simulink model "test"  (R2022a)
settings: Solver=VariableStepAuto  StartTime=0.0  StopTime=30  RelTol=1e-3
values from neighbouring files (symbols this model uses):
  n = length(stations)    [ethernetHubMask.m]
undefined symbols (not defined in the file or in its folder): gateControl, m, networkselector
settings Model: Creator=lch  LastModifiedBy=lch

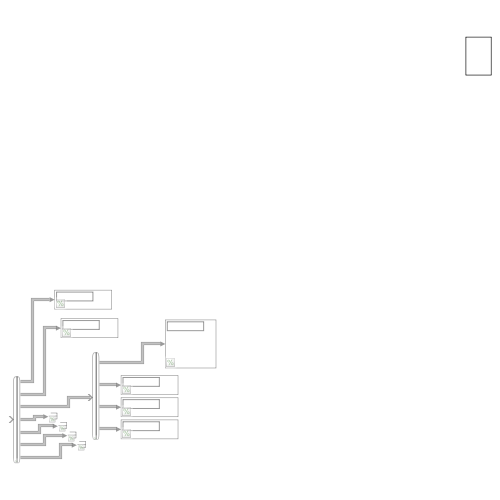
[thumbnail: Simulink's stored preview of the top-level diagram]
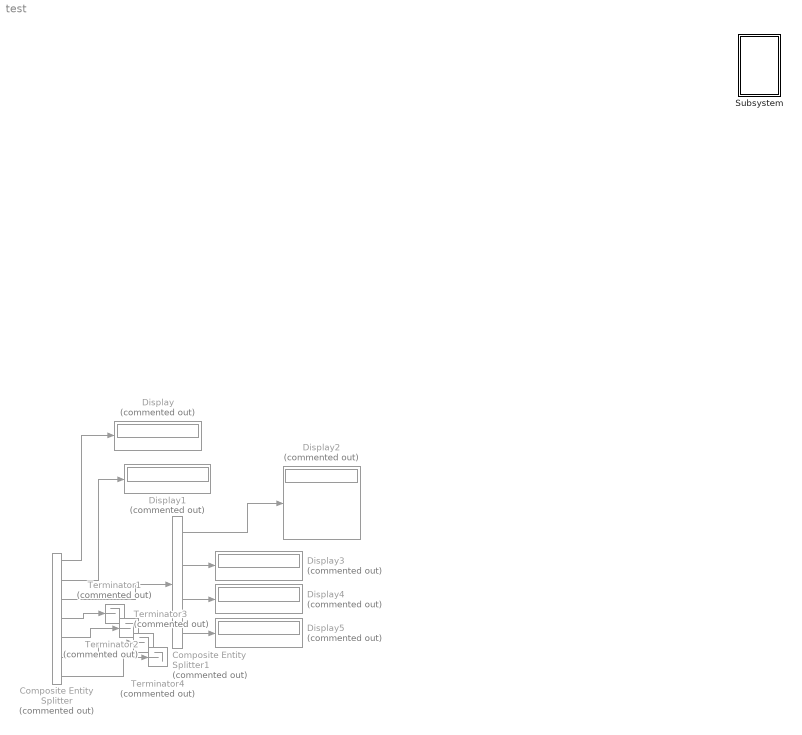
== system test ==
  Composite Entity Splitter : CompositeEntitySplitter  Commented=on  InputPortMessageModes=m  OutputPortMessageModes=m,m,m,m,m,m,m  NumberOutputPorts=7
      settings: OutputPortMap=o0,o1,o2,o3,o4,o5,o6
  Composite Entity Splitter1 : CompositeEntitySplitter  Commented=on  InputPortMessageModes=m  OutputPortMessageModes=m,m,m,m  NumberOutputPorts=4
      settings: OutputPortMap=o0,o1,o2,o3
  Display{,1..5} (6 alike) : Display  Commented=on
  Subsystem : Subsystem
  Terminator{1..4} (4 alike) : Terminator  Commented=on
  wires:
  Composite Entity Splitter/1 -> Display/1
  Composite Entity Splitter/2 -> Display1/1
  Composite Entity Splitter/3 -> Composite Entity Splitter1/1
  Composite Entity Splitter/4 -> Terminator1/1
  Composite Entity Splitter/5 -> Terminator2/1
  Composite Entity Splitter/6 -> Terminator3/1
  Composite Entity Splitter/7 -> Terminator4/1
  Composite Entity Splitter1/1 -> Display2/1
  Composite Entity Splitter1/2 -> Display3/1
  Composite Entity Splitter1/3 -> Display4/1
  Composite Entity Splitter1/4 -> Display5/1

== system test/Subsystem ==
  Subsystem : Subsystem  mask{ip=[10 1 2 1]}
      mask prompts: ip "IP Address"
      mask DialogControl ParameterGroupVar Prompt: 파라미터

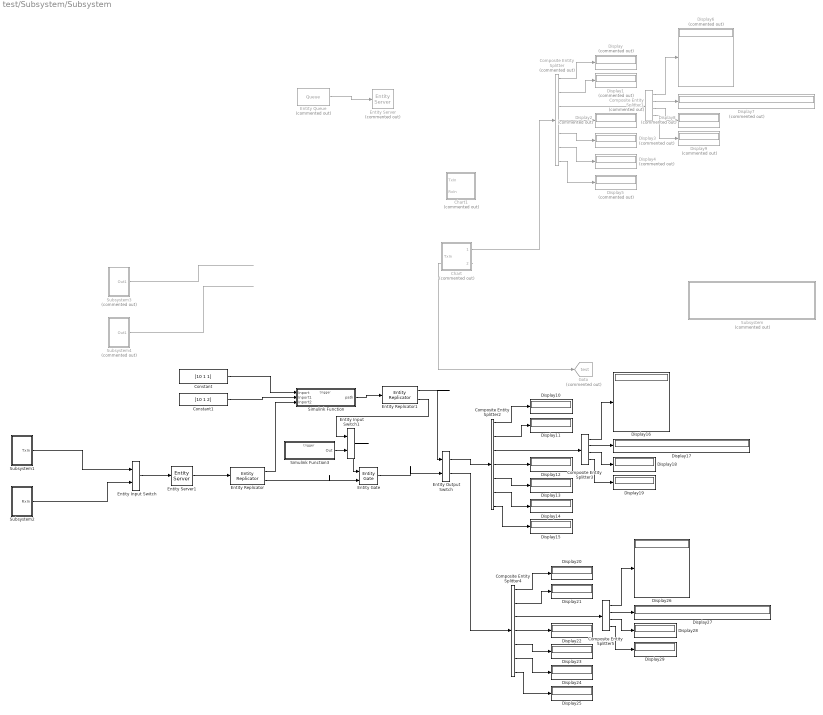
== system test/Subsystem/Subsystem ==
  Chart : Stateflow chart  Commented=on  TreatAsAtomicUnit=on
  Chart1 : Stateflow chart  Commented=on  TreatAsAtomicUnit=on
  Composite Entity Splitter : CompositeEntitySplitter  Commented=on  InputPortMessageModes=m  OutputPortMessageModes=m,m,m,m,m,m,m  NumberOutputPorts=7
      settings: OutputPortMap=o0,o1,o2,o3,o4,o5,o6
  Composite Entity Splitter1 : CompositeEntitySplitter  Commented=on  InputPortMessageModes=m  OutputPortMessageModes=m,m,m,m  NumberOutputPorts=4
      settings: OutputPortMap=o0,o1,o2,o3
  Composite Entity Splitter2 : CompositeEntitySplitter  InputPortMessageModes=m  OutputPortMessageModes=m,m,m,m,m,m,m  NumberOutputPorts=7
      settings: OutputPortMap=o0,o1,o2,o3,o4,o5,o6
  Composite Entity Splitter3 : CompositeEntitySplitter  InputPortMessageModes=m  OutputPortMessageModes=m,m,m,m  NumberOutputPorts=4
      settings: OutputPortMap=o0,o1,o2,o3
  Composite Entity Splitter4 : CompositeEntitySplitter  InputPortMessageModes=m  OutputPortMessageModes=m,m,m,m,m,m,m  NumberOutputPorts=7
      settings: OutputPortMap=o0,o1,o2,o3,o4,o5,o6
  Composite Entity Splitter5 : CompositeEntitySplitter  InputPortMessageModes=m  OutputPortMessageModes=m,m,m,m  NumberOutputPorts=4
      settings: OutputPortMap=o0,o1,o2,o3
  Constant : Constant  Value=[10 1 1]
  Constant1 : Constant  Value=[10 1 2]
  Display{,1..9} (10 alike) : Display  Commented=on
  Display{10..29} (20 alike) : Display
  Entity Input Switch : EntityInputSwitch  InputPortMessageModes=m,m  OutputPortMessageModes=m
  Entity Input Switch1 : EntityInputSwitch  InputPortMessageModes=m,m  OutputPortMessageModes=m
  Entity Output Switch : EntityOutputSwitch  InputPortMessageModes=m,m  OutputPortMessageModes=m,m  SwitchingCriterion=From control port  SwitchAttributeName=Attribute1
      settings: InputPortMap=u0,u1
  Entity Gate : EntityGate  InputPortMessageModes=m,m  OutputPortMessageModes=m  OpenGateAtSimulationStart=on
  Entity Queue : Queue  Commented=on  InputPortMessageModes=m  OutputPortMessageModes=m  Capacity=255
  Entity Replicator : EntityReplicator  InputPortMessageModes=m  OutputPortMessageModes=m,m
  Entity Replicator1 : EntityReplicator  InputPortMessageModes=m  OutputPortMessageModes=m,m
  Entity Server : EntityServer  Commented=on  InputPortMessageModes=m  OutputPortMessageModes=m  Capacity=255  ServiceTimeValue=0.01
  Entity Server1 : EntityServer  InputPortMessageModes=m  OutputPortMessageModes=m  Capacity=inf  ServiceTimeSource=MATLAB action  ServiceCompleteAction=networkselector();  ExitAction=gateControl();
  Goto : Goto  Commented=on  GotoTag=test  TagVisibility=global
  Simulink Function : Subsystem  TreatAsAtomicUnit=on
  Simulink Function3 : Subsystem  TreatAsAtomicUnit=on
  Subsystem : Subsystem  Commented=on  mask{vlan1=[10 1 3], vlan2=[10 1 4]}
      mask DialogControl ParameterGroupVar Prompt: 파라미터
  Subsystem1 : Subsystem
  Subsystem2 : Subsystem
  Subsystem3 : Subsystem  Commented=on
  Subsystem4 : Subsystem  Commented=on
  wires:
  Composite Entity Splitter/1 -> Display/1
  Composite Entity Splitter/2 -> Display1/1
  Composite Entity Splitter/3 -> Composite Entity Splitter1/1
  Composite Entity Splitter/4 -> Display2/1
  Composite Entity Splitter/5 -> Display3/1
  Composite Entity Splitter/6 -> Display4/1
  Composite Entity Splitter/7 -> Display5/1
  Composite Entity Splitter1/1 -> Display6/1
  Composite Entity Splitter1/2 -> Display7/1
  Composite Entity Splitter1/3 -> Display8/1
  Composite Entity Splitter1/4 -> Display9/1
  Chart/1(LocalNet) -> Composite Entity Splitter/1
  Chart/2(OtherNet) -> Goto/1
  Subsystem3/1(Out1) -> ?
  Subsystem4/1(Out1) -> ?
  Entity Queue/1 -> Entity Server/1
  Subsystem1/1(TxIn) -> Entity Input Switch/1
  Subsystem2/1(RxIn) -> Entity Input Switch/2
  Entity Input Switch/1 -> Entity Server1/1
  Constant/1 -> Simulink Function/1(Inport)
  Constant1/1 -> Simulink Function/2(Inport1)
  Simulink Function/1(path) -> Entity Replicator1/1
  Composite Entity Splitter3/4 -> Display19/1
  Composite Entity Splitter2/3 -> Composite Entity Splitter3/1
  Composite Entity Splitter3/3 -> Display18/1
  Composite Entity Splitter2/4 -> Display12/1
  Composite Entity Splitter2/7 -> Display15/1
  Composite Entity Splitter2/6 -> Display14/1
  Composite Entity Splitter3/2 -> Display17/1
  Composite Entity Splitter3/1 -> Display16/1
  Composite Entity Splitter2/5 -> Display13/1
  Composite Entity Splitter2/2 -> Display11/1
  Composite Entity Splitter2/1 -> Display10/1
  Entity Output Switch/1 -> Composite Entity Splitter2/1
  Composite Entity Splitter5/4 -> Display29/1
  Composite Entity Splitter4/3 -> Composite Entity Splitter5/1
  Composite Entity Splitter5/3 -> Display28/1
  Composite Entity Splitter4/4 -> Display22/1
  Composite Entity Splitter4/7 -> Display25/1
  Composite Entity Splitter4/6 -> Display24/1
  Composite Entity Splitter5/2 -> Display27/1
  Composite Entity Splitter5/1 -> Display26/1
  Composite Entity Splitter4/5 -> Display23/1
  Composite Entity Splitter4/2 -> Display21/1
  Composite Entity Splitter4/1 -> Display20/1
  Entity Output Switch/2 -> Composite Entity Splitter4/1
  Entity Replicator1/2 -> Entity Input Switch1/1
  Entity Replicator1/1 -> Entity Output Switch/1
  Entity Gate/1 -> Entity Output Switch/2
  Entity Input Switch1/1 -> Entity Gate/1
  Simulink Function3/1(Out) -> Entity Input Switch1/2
  Entity Server1/1 -> Entity Replicator/1
  Entity Replicator/1 -> Simulink Function/3(Inport2)
  Entity Replicator/2 -> Entity Gate/2

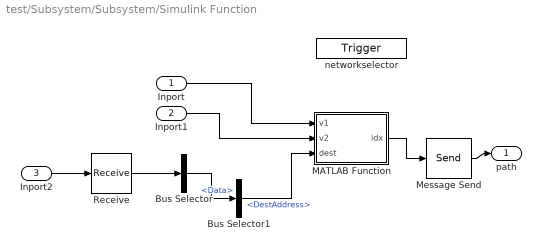
== system test/Subsystem/Subsystem/Simulink Function ==
  Inport : Inport
  Inport1 : Inport  Port=2
  Inport2 : Inport  Port=3
  networkselector : TriggerPort  TriggerType=function-call  IsSimulinkFunction=on  FunctionName=networkselector  FunctionVisibility=scoped  VariantControl=(inherit)
  Bus Selector : BusSelector  OutputSignals=Data
  Bus Selector1 : BusSelector  OutputSignals=DestAddress
  MATLAB Function : MATLAB Function  TreatAsAtomicUnit=on
  Message Send : Send  OutputPortMessageModes=m
  Receive : Receive  InputPortMessageModes=m  UseInternalQueue=off  QueueOverwriting=on  QueueLength=1  QueueType=LIFO
  path : Outport
  wires:
  Receive/1 -> Bus Selector/1
  Inport/1 -> MATLAB Function/1(v1)
  Inport1/1 -> MATLAB Function/2(v2)
  Bus Selector/1 -> Bus Selector1/1  "<Data>"
  MATLAB Function/1(idx) -> Message Send/1
  Message Send/1 -> path/1
  Inport2/1 -> Receive/1
  Bus Selector1/1 -> MATLAB Function/3(dest)  "<DestAddress>"

== system test/Subsystem/Subsystem/Simulink Function3 ==
  gateControl : TriggerPort  TriggerType=function-call  IsSimulinkFunction=on  FunctionName=gateControl  FunctionVisibility=scoped  VariantControl=Variant
  Constant : Constant  Value=0
  Message Send : Send  OutputPortMessageModes=m
  Out : Outport
  wires:
  Message Send/1 -> Out/1
  Constant/1 -> Message Send/1

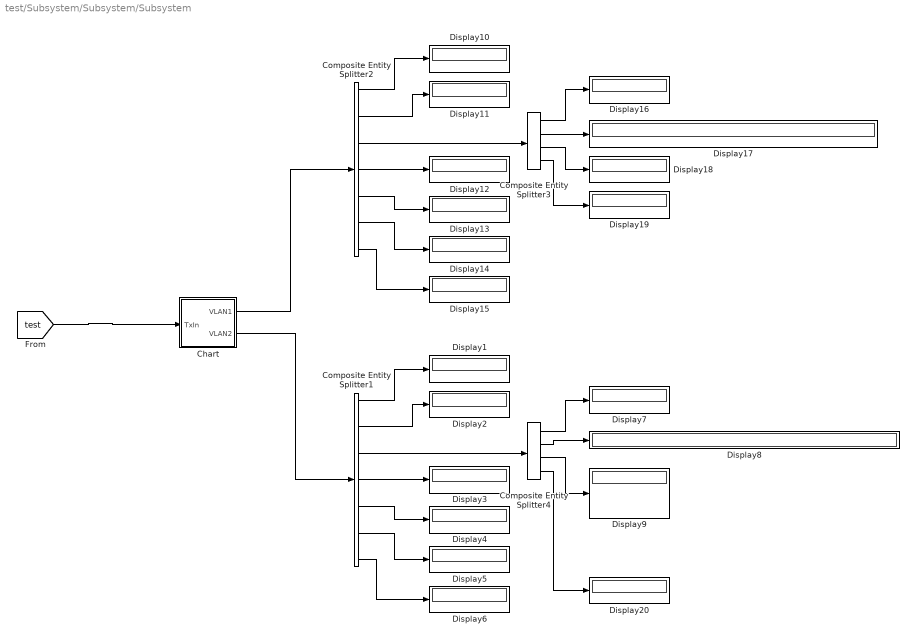
== system test/Subsystem/Subsystem/Subsystem ==
  Chart : Stateflow chart  TreatAsAtomicUnit=on
  Composite Entity Splitter1 : CompositeEntitySplitter  InputPortMessageModes=m  OutputPortMessageModes=m,m,m,m,m,m,m  NumberOutputPorts=7
      settings: OutputPortMap=o0,o1,o2,o3,o4,o5,o6
  Composite Entity Splitter2 : CompositeEntitySplitter  InputPortMessageModes=m  OutputPortMessageModes=m,m,m,m,m,m,m  NumberOutputPorts=7
      settings: OutputPortMap=o0,o1,o2,o3,o4,o5,o6
  Composite Entity Splitter3 : CompositeEntitySplitter  InputPortMessageModes=m  OutputPortMessageModes=m,m,m,m  NumberOutputPorts=4
      settings: OutputPortMap=o0,o1,o2,o3
  Composite Entity Splitter4 : CompositeEntitySplitter  InputPortMessageModes=m  OutputPortMessageModes=m,m,m,m  NumberOutputPorts=4
      settings: OutputPortMap=o0,o1,o2,o3
  Display{1..20} (20 alike) : Display
  wires:
  [test] -> Chart/1(TxIn)
  Composite Entity Splitter3/4 -> Display19/1
  Composite Entity Splitter2/3 -> Composite Entity Splitter3/1
  Composite Entity Splitter2/5 -> Display13/1
  Composite Entity Splitter2/6 -> Display14/1
  Composite Entity Splitter2/2 -> Display11/1
  Composite Entity Splitter2/7 -> Display15/1
  Composite Entity Splitter3/1 -> Display16/1
  Composite Entity Splitter3/2 -> Display17/1
  Composite Entity Splitter3/3 -> Display18/1
  Composite Entity Splitter2/1 -> Display10/1
  Composite Entity Splitter2/4 -> Display12/1
  Chart/1(VLAN1) -> Composite Entity Splitter2/1
  Composite Entity Splitter1/1 -> Display1/1
  Composite Entity Splitter4/3 -> Display9/1
  Composite Entity Splitter4/1 -> Display7/1
  Composite Entity Splitter1/5 -> Display4/1
  Composite Entity Splitter1/3 -> Composite Entity Splitter4/1
  Composite Entity Splitter1/4 -> Display3/1
  Composite Entity Splitter4/2 -> Display8/1
  Composite Entity Splitter1/7 -> Display6/1
  Composite Entity Splitter1/2 -> Display2/1
  Composite Entity Splitter4/4 -> Display20/1
  Composite Entity Splitter1/6 -> Display5/1
  Chart/2(VLAN2) -> Composite Entity Splitter1/1

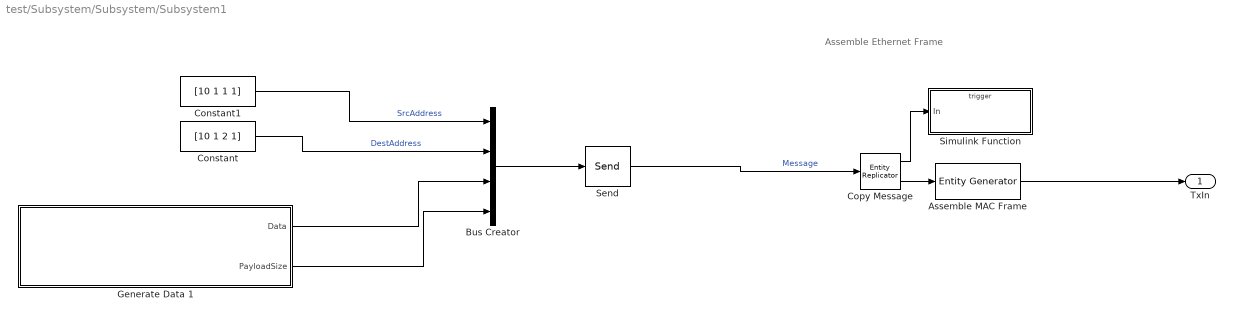
== system test/Subsystem/Subsystem/Subsystem1 ==
  note: Assemble Ethernet Frame
  Assemble MAC Frame : EntityGenerator  InputPortMessageModes=m  OutputPortMessageModes=m  GenerationMethod=Event-based  GenerateAction=|  EntityType=Bus object  EntityTypeName=ethernetPacket
      | entity.TxAddress = 1;
      | entity.RxAddress = 0;
      | [entity.Data, entity.PayloadSize] = initPacket();
      | entity.TxDelay = (entity.PayloadSize+22)*8/BitRate;
      | entity.BackoffTime = 0;
      | entity.CRC = 0;
      settings: InputPortMap=u0
  Bus Creator : BusCreator  Inputs=4  OutDataTypeStr=Bus: dataPacket  NonVirtualBus=on
  Constant : Constant  Value=[10 1 2 1]
  Constant1 : Constant  Value=[10 1 1 1]
  Copy Message : EntityReplicator  InputPortMessageModes=m  OutputPortMessageModes=m,m
  Generate Data 1 : MATLAB Function  TreatAsAtomicUnit=on  SystemSampleTime=0.01
  Send : Send  OutputPortMessageModes=m
  Simulink Function : Subsystem  TreatAsAtomicUnit=on
  TxIn : Outport
  wires:
  Copy Message/2 -> Assemble MAC Frame/1
  Generate Data 1/1(Data) -> Bus Creator/3
  Send/1 -> Copy Message/1  "Message"
  Constant1/1 -> Bus Creator/1  "SrcAddress"
  Bus Creator/1 -> Send/1
  Copy Message/1 -> Simulink Function/1(In)
  Constant/1 -> Bus Creator/2  "DestAddress"
  Generate Data 1/2(PayloadSize) -> Bus Creator/4
  Assemble MAC Frame/1 -> TxIn/1

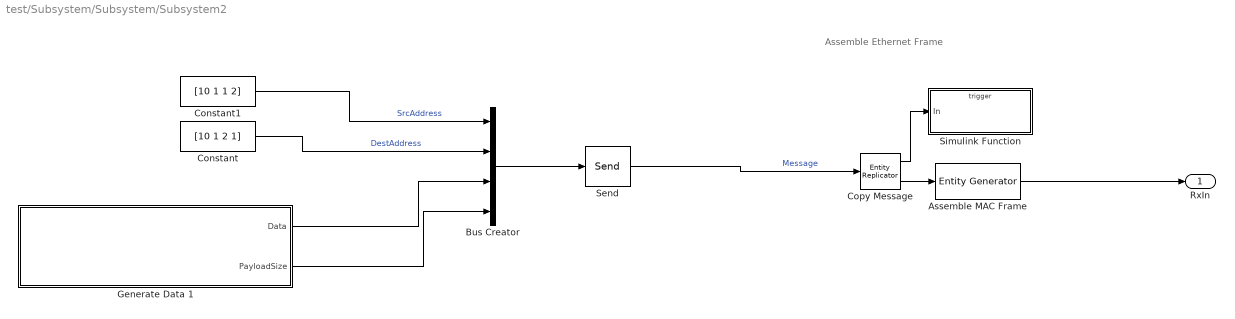
== system test/Subsystem/Subsystem/Subsystem2 ==
  note: Assemble Ethernet Frame
  Assemble MAC Frame : EntityGenerator  InputPortMessageModes=m  OutputPortMessageModes=m  GenerationMethod=Event-based  GenerateAction=|  EntityType=Bus object  EntityTypeName=ethernetPacket
      | entity.TxAddress = 1;
      | entity.RxAddress = 0;
      | [entity.Data, entity.PayloadSize] = initPacket();
      | entity.TxDelay = (entity.PayloadSize+22)*8/BitRate;
      | entity.BackoffTime = 0;
      | entity.CRC = 0;
      settings: InputPortMap=u0
  Bus Creator : BusCreator  Inputs=4  OutDataTypeStr=Bus: dataPacket  NonVirtualBus=on
  Constant : Constant  Value=[10 1 2 1]
  Constant1 : Constant  Value=[10 1 1 2]
  Copy Message : EntityReplicator  InputPortMessageModes=m  OutputPortMessageModes=m,m
  Generate Data 1 : MATLAB Function  TreatAsAtomicUnit=on  SystemSampleTime=0.01
  Send : Send  OutputPortMessageModes=m
  Simulink Function : Subsystem  TreatAsAtomicUnit=on
  RxIn : Outport
  wires:
  Assemble MAC Frame/1 -> RxIn/1
  Generate Data 1/2(PayloadSize) -> Bus Creator/4
  Constant/1 -> Bus Creator/2  "DestAddress"
  Copy Message/1 -> Simulink Function/1(In)
  Bus Creator/1 -> Send/1
  Constant1/1 -> Bus Creator/1  "SrcAddress"
  Send/1 -> Copy Message/1  "Message"
  Generate Data 1/1(Data) -> Bus Creator/3
  Copy Message/2 -> Assemble MAC Frame/1

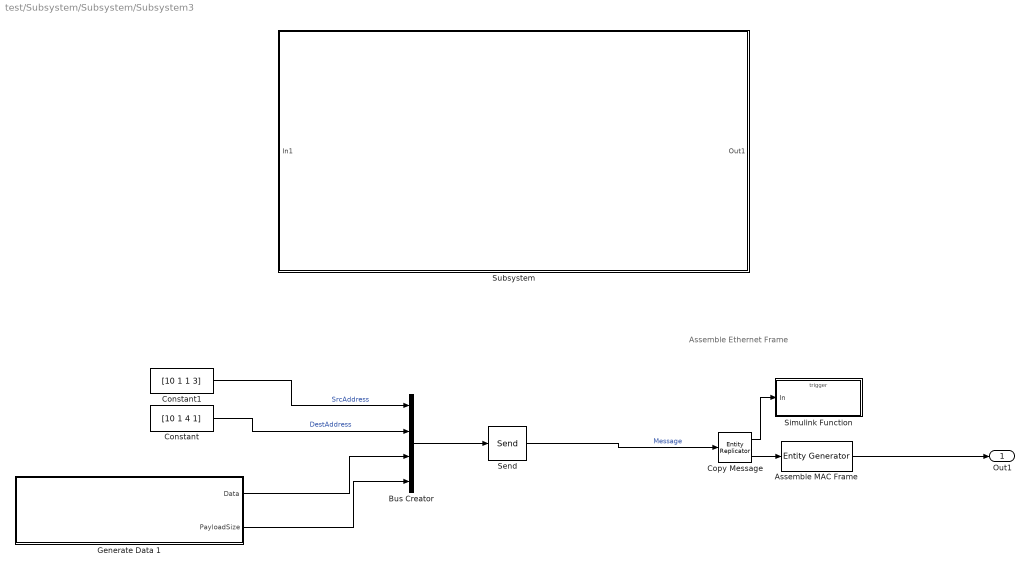
== system test/Subsystem/Subsystem/Subsystem3 ==
  note: Assemble Ethernet Frame
  Assemble MAC Frame : EntityGenerator  InputPortMessageModes=m  OutputPortMessageModes=m  GenerationMethod=Event-based  GenerateAction=|  EntityType=Bus object  EntityTypeName=ethernetPacket
      | entity.TxAddress = 1;
      | entity.RxAddress = 0;
      | [entity.Data, entity.PayloadSize] = initPacket();
      | entity.TxDelay = (entity.PayloadSize+22)*8/BitRate;
      | entity.BackoffTime = 0;
      | entity.CRC = 0;
      settings: InputPortMap=u0
  Bus Creator : BusCreator  Inputs=4  OutDataTypeStr=Bus: dataPacket  NonVirtualBus=on
  Constant : Constant  Value=[10 1 4 1]
  Constant1 : Constant  Value=[10 1 1 3]
  Copy Message : EntityReplicator  InputPortMessageModes=m  OutputPortMessageModes=m,m
  Generate Data 1 : MATLAB Function  TreatAsAtomicUnit=on  SystemSampleTime=0.2
  Send : Send  OutputPortMessageModes=m
  Simulink Function : Subsystem  TreatAsAtomicUnit=on
  Subsystem : Subsystem
  Out1 : Outport
  wires:
  Copy Message/2 -> Assemble MAC Frame/1
  Generate Data 1/1(Data) -> Bus Creator/3
  Send/1 -> Copy Message/1  "Message"
  Constant1/1 -> Bus Creator/1  "SrcAddress"
  Bus Creator/1 -> Send/1
  Copy Message/1 -> Simulink Function/1(In)
  Constant/1 -> Bus Creator/2  "DestAddress"
  Generate Data 1/2(PayloadSize) -> Bus Creator/4
  Assemble MAC Frame/1 -> Out1/1

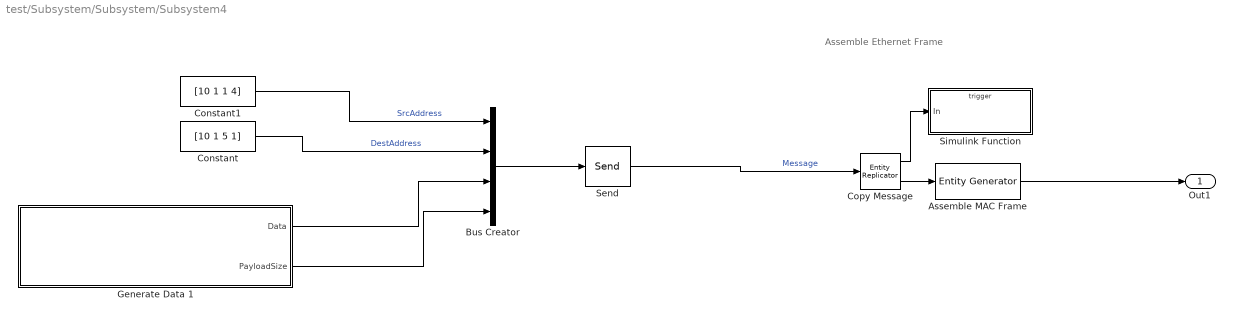
== system test/Subsystem/Subsystem/Subsystem4 ==
  note: Assemble Ethernet Frame
  Assemble MAC Frame : EntityGenerator  InputPortMessageModes=m  OutputPortMessageModes=m  GenerationMethod=Event-based  GenerateAction=|  EntityType=Bus object  EntityTypeName=ethernetPacket
      | entity.TxAddress = 1;
      | entity.RxAddress = 0;
      | [entity.Data, entity.PayloadSize] = initPacket();
      | entity.TxDelay = (entity.PayloadSize+22)*8/BitRate;
      | entity.BackoffTime = 0;
      | entity.CRC = 0;
      settings: InputPortMap=u0
  Bus Creator : BusCreator  Inputs=4  OutDataTypeStr=Bus: dataPacket  NonVirtualBus=on
  Constant : Constant  Value=[10 1 5 1]
  Constant1 : Constant  Value=[10 1 1 4]
  Copy Message : EntityReplicator  InputPortMessageModes=m  OutputPortMessageModes=m,m
  Generate Data 1 : MATLAB Function  TreatAsAtomicUnit=on  SystemSampleTime=0.2
  Send : Send  OutputPortMessageModes=m
  Simulink Function : Subsystem  TreatAsAtomicUnit=on
  Out1 : Outport
  wires:
  Assemble MAC Frame/1 -> Out1/1
  Generate Data 1/2(PayloadSize) -> Bus Creator/4
  Constant/1 -> Bus Creator/2  "DestAddress"
  Copy Message/1 -> Simulink Function/1(In)
  Bus Creator/1 -> Send/1
  Constant1/1 -> Bus Creator/1  "SrcAddress"
  Send/1 -> Copy Message/1  "Message"
  Generate Data 1/1(Data) -> Bus Creator/3
  Copy Message/2 -> Assemble MAC Frame/1

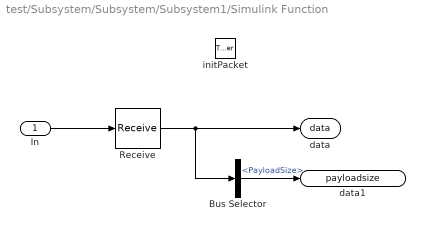
== system test/Subsystem/Subsystem/Subsystem1/Simulink Function ==
  In : Inport
  initPacket : TriggerPort  TriggerType=function-call  IsSimulinkFunction=on  FunctionName=initPacket  FunctionVisibility=scoped  VariantControl=(inherit)
  Bus Selector : BusSelector  OutputSignals=PayloadSize
  Receive : Receive  InputPortMessageModes=m  QueueLength=2^16-1
  data : ArgOut  DisableCoverage=on  OutDataTypeStr=Bus: dataPacket  ArgumentName=data
  data1 : ArgOut  DisableCoverage=on  Port=2  ArgumentName=payloadsize
  wires:
  Receive/1 -> Bus Selector/1, data/1
  In/1 -> Receive/1
  Bus Selector/1 -> data1/1  "<PayloadSize>"

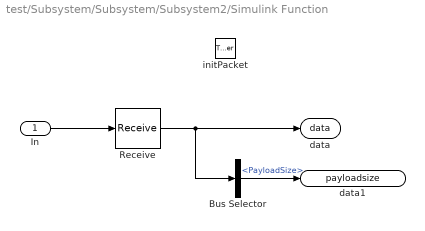
== system test/Subsystem/Subsystem/Subsystem2/Simulink Function ==
  In : Inport
  initPacket : TriggerPort  TriggerType=function-call  IsSimulinkFunction=on  FunctionName=initPacket  FunctionVisibility=scoped  VariantControl=(inherit)
  Bus Selector : BusSelector  OutputSignals=PayloadSize
  Receive : Receive  InputPortMessageModes=m  QueueLength=2^16-1
  data : ArgOut  DisableCoverage=on  OutDataTypeStr=Bus: dataPacket  ArgumentName=data
  data1 : ArgOut  DisableCoverage=on  Port=2  ArgumentName=payloadsize
  wires:
  Bus Selector/1 -> data1/1  "<PayloadSize>"
  In/1 -> Receive/1
  Receive/1 -> data/1, Bus Selector/1

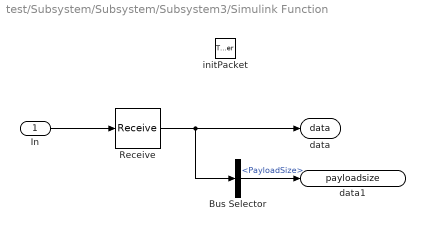
== system test/Subsystem/Subsystem/Subsystem3/Simulink Function ==
  In : Inport
  initPacket : TriggerPort  TriggerType=function-call  IsSimulinkFunction=on  FunctionName=initPacket  FunctionVisibility=scoped  VariantControl=(inherit)
  Bus Selector : BusSelector  OutputSignals=PayloadSize
  Receive : Receive  InputPortMessageModes=m  QueueLength=2^16-1
  data : ArgOut  DisableCoverage=on  OutDataTypeStr=Bus: dataPacket  ArgumentName=data
  data1 : ArgOut  DisableCoverage=on  Port=2  ArgumentName=payloadsize
  wires:
  Receive/1 -> Bus Selector/1, data/1
  In/1 -> Receive/1
  Bus Selector/1 -> data1/1  "<PayloadSize>"

== system test/Subsystem/Subsystem/Subsystem3/Subsystem ==
  In1 : Inport
  Out1 : Outport
  wires:
  In1/1 -> Out1/1

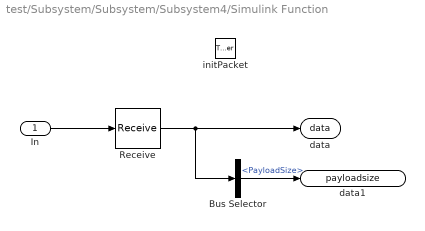
== system test/Subsystem/Subsystem/Subsystem4/Simulink Function ==
  In : Inport
  initPacket : TriggerPort  TriggerType=function-call  IsSimulinkFunction=on  FunctionName=initPacket  FunctionVisibility=scoped  VariantControl=(inherit)
  Bus Selector : BusSelector  OutputSignals=PayloadSize
  Receive : Receive  InputPortMessageModes=m  QueueLength=2^16-1
  data : ArgOut  DisableCoverage=on  OutDataTypeStr=Bus: dataPacket  ArgumentName=data
  data1 : ArgOut  DisableCoverage=on  Port=2  ArgumentName=payloadsize
  wires:
  Bus Selector/1 -> data1/1  "<PayloadSize>"
  In/1 -> Receive/1
  Receive/1 -> data/1, Bus Selector/1

== matlab function test/Subsystem/Subsystem/Subsystem3/Generate Data 1 ==
  data: Data output; PayloadSize output
function [Data, PayloadSize] = randomLengthPayload()
% Generate Ethernet payload of random length between min and max frame size
PayloadSize = 45+randi(1455); % Payload length is 46-1500 bytes
Data = zeros(1,1500);
Data(1:PayloadSize) = randi(256,1, PayloadSize)-1; % Payload values are random (0-255) for a byte

== matlab function test/Subsystem/Subsystem/Subsystem4/Generate Data 1 ==
  data: Data output; PayloadSize output
function [Data, PayloadSize] = randomLengthPayload()
% Generate Ethernet payload of random length between min and max frame size
PayloadSize = 45+randi(1455); % Payload length is 46-1500 bytes
Data = zeros(1,1500);
Data(1:PayloadSize) = randi(256,1, PayloadSize)-1; % Payload values are random (0-255) for a byte

== stateflow chart test/Subsystem/Subsystem/Chart1 ==
  state B
    en:
    log.data = TxIn.data.Data.DestAddress
  state init
  state A
  state K
    en:
    log.data=RxIn.data.Data.DestAddress
  state sus
    en:
    log.data=[0 0 0 0]
  B -> init
  (default) -> init
  A -> B [order 1] : TxIn[TxIn.data.Data.DestAddress(3)==2]
  init -> A [order 1] : TxIn
  sus -> init
  K -> init
  init -> K [order 2] : RxIn
  A -> sus [order 2] : after(0.0002,sec)
  data: TxIn input Bus: ethernetPacket; log local double; RxIn input Bus: ethernetPacket

== matlab function test/Subsystem/Subsystem/Simulink Function/MATLAB Function ==
  data: v1 input; idx output; v2 input; dest input
function idx = fcn(v1,v2,dest)

if(v1(1)==dest(1)&&v1(2)==dest(2)&&v1(3)==dest(3))
    idx=1;
elseif(v2(1)==dest(1)&&v2(2)==dest(2)&&v2(3)==dest(3))
    idx=2;
else
    idx=1;
end

== matlab function test/Subsystem/Subsystem/Subsystem1/Generate Data 1 ==
  data: Data output; PayloadSize output
function [Data, PayloadSize] = randomLengthPayload()
% Generate Ethernet payload of random length between min and max frame size
PayloadSize = 45+randi(1455); % Payload length is 46-1500 bytes
Data = zeros(1,1500);
Data(1:PayloadSize) = randi(256,1, PayloadSize)-1; % Payload values are random (0-255) for a byte

== stateflow chart test/Subsystem/Subsystem/Subsystem/Chart ==
  state Init
  state VLANInspec
    en:
    DestAddress = TxIn.data.Data.DestAddress;
  state V1
    en:
    send(VLAN1);
  state V2
    en:
    send(VLAN2);
  (default) -> Init
  V2 -> Init
  V1 -> Init
  Init -> VLANInspec : TxIn
  VLANInspec -> V2 [order 2] : TxIn[DestAddress(1)==vlan2(1) ...
      |     && DestAddress(2)==vlan2(2)...
      |     && DestAddress(3)==vlan2(3)]{VLAN2.data=TxIn.data;}
  VLANInspec -> V1 [order 1] : TxIn[DestAddress(1)==vlan1(1) ...
      |     && DestAddress(2)==vlan1(2)...
      |     && DestAddress(3)==vlan1(3)]{VLAN1.data=TxIn.data;}
  data: TxIn input Bus: ethernetPacket size=1; VLAN1 output Bus: ethernetPacket size=1; VLAN2 output Bus: ethernetPacket size=1; DestAddress local; vlan2 parameter; vlan1 parameter

== stateflow chart test/Subsystem/Subsystem/Chart ==
  state Stanby
    en:
    NetAddress = ip(1:3);
  state NetInspec
    en:
    DestAddress = TxIn.data.Data.DestAddress;
  state DiffNetAddress
    en:
    send(OtherNet);
  state SameNetAddress
    en:
    send(LocalNet);
  (default) -> Stanby
  DiffNetAddress -> Stanby
  SameNetAddress -> Stanby
  Stanby -> NetInspec : TxIn
  NetInspec -> SameNetAddress [order 2] : TxIn[DestAddress(1)==NetAddress(1) ...
      |     && DestAddress(2)==NetAddress(2)...
      |     && DestAddress(3)==NetAddress(3)]{LocalNet.data=TxIn.data;}
  NetInspec -> DiffNetAddress [order 1] : TxIn{OtherNet.data=TxIn.data;}
  data: TxIn input Bus: ethernetPacket size=1; ip parameter; NetAddress local; LocalNet output Bus: ethernetPacket size=1; OtherNet output Bus: ethernetPacket size=1; DestAddress local

== matlab function test/Subsystem/Subsystem/Subsystem2/Generate Data 1 ==
  data: Data output; PayloadSize output
function [Data, PayloadSize] = randomLengthPayload()
% Generate Ethernet payload of random length between min and max frame size
PayloadSize = 45+randi(1455); % Payload length is 46-1500 bytes
Data = zeros(1,1500);
Data(1:PayloadSize) = randi(256,1, PayloadSize)-1; % Payload values are random (0-255) for a byte
